simulink model "mconversionOtherInstanceBuses"  (Simulink 8.0)
settings: Solver=FixedStepDiscrete  StartTime=0.0  StopTime=10.0  RelTol=1e-3
libraries: busLib x4, simulink x1
settings Model: Creator=awarlock  LastModifiedBy=htu  ExtModeAutoUpdateStatusClock=off
settings DataIOCC: SignalLoggingSaveFormat=ModelDataLogs
settings OptimizationCC: InlineParams=on  InlineInvariantSignals=on  InitFltsAndDblsToZero=on
settings DebuggingCC: SaveWithParameterizedLinksMsg=none  SignalResolutionControl=TryResolveAllWithWarning  MultiTaskDSMMsg=warning  MultiTaskCondExecSysMsg=none
settings RTWCC: IncludeERTFirstTime=on
settings GRTTargetCC: TargetFcnLib=ansi_tfl_tmw.mat  CombineOutputUpdateFcns=off  GRTInterface=on

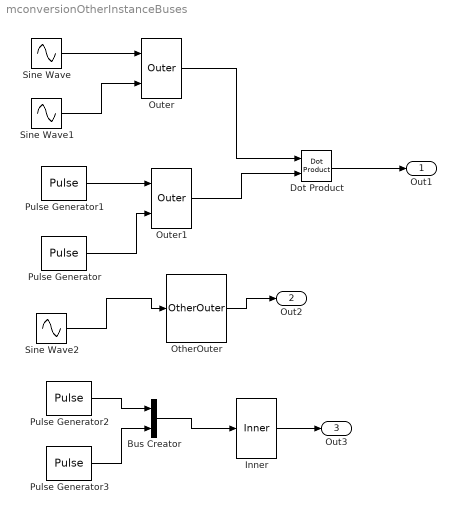
== system mconversionOtherInstanceBuses ==
  Bus Creator : BusCreator  DialogController=Simulink.DDGSource_Bus  Inputs=2
  Dot Product : simulink/Math Operations/Dot Product  InputSameDT=on  OutDataType=sfix(16)  OutScaling=2^-10  DoSatur=off
  Inner : busLib/Inner
  OtherOuter : busLib/OtherOuter
  Outer : busLib/Outer
  Outer1 : busLib/Outer
  Pulse Generator : DiscretePulseGenerator  SampleTime=0.1
  Pulse Generator1 : DiscretePulseGenerator  SampleTime=0.1
  Pulse Generator2 : DiscretePulseGenerator  Amplitude=5  SampleTime=0.1
  Pulse Generator3 : DiscretePulseGenerator  Period=5  PulseWidth=3  SampleTime=0.1
  Sine Wave : Sin  SampleTime=0.1
  Sine Wave1 : Sin  SampleTime=0.1
  Sine Wave2 : Sin  Phase=0.5  SampleTime=0.1
  Out1 : Outport
  Out2 : Outport  Port=2
  Out3 : Outport  Port=3
  wires:
  Sine Wave/1 -> Outer/1
  Sine Wave1/1 -> Outer/2
  Pulse Generator1/1 -> Outer1/1
  Pulse Generator/1 -> Outer1/2
  Outer/1 -> Dot Product/1
  Outer1/1 -> Dot Product/2
  Dot Product/1 -> Out1/1
  Sine Wave2/1 -> OtherOuter/1
  OtherOuter/1 -> Out2/1
  Pulse Generator2/1 -> Bus Creator/1
  Pulse Generator3/1 -> Bus Creator/2
  Bus Creator/1 -> Inner/1
  Inner/1 -> Out3/1
